simulink model "Wind_Harness"  (R2025b)
settings: Solver=VariableStepAuto  StartTime=0.0  StopTime=5  FixedStep=5e-5  RelTol=1e-3
PostLoadFcn:
  | WindFarmParam;
values from neighbouring files (symbols this model uses):
  base = struct    [WindFarmParam.m]
  pmsm = struct    [WindFarmParam.m]
  Ts = 5E-5    (= 5e-05)    [BESSGFLParam.m]    (also in BESSGFMParam.m; WindFarmParam.m)
  windController = struct    [WindFarmParam.m]
  windSystem = struct    [WindFarmParam.m]
  windTurbine = saveVarsMat.windTurbine    [WindFarmParam.m]
undefined symbols (not defined in the file or in its folder): DiscIntNeverNeededParam, Inertia
libraries: nesl_utility x34, fl_lib x18, ee_lib x18, eeTransforms x6, eeGeneralControl x5, simulink x4, eePwmGenerator x2, eeSinusoidalMeasurementV2 x1, eePmsmCurrentController x1, custom_lib x1
(part 1 of 2)
settings Model: SimulationMode=accelerator  Creator=skota  LastModifiedBy=skota

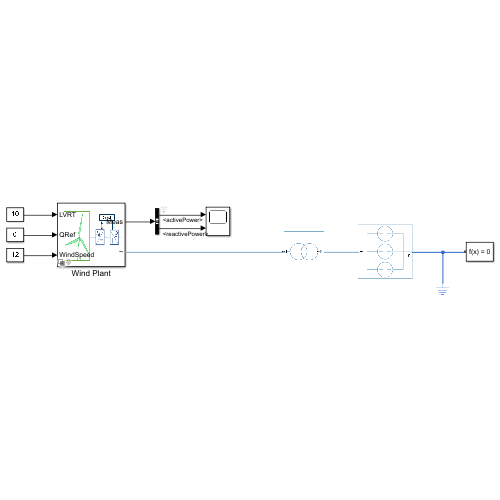
[thumbnail: Simulink's stored preview of the top-level diagram]
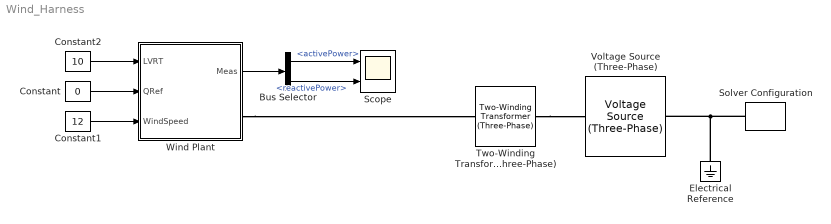
== system Wind_Harness ==
  Bus Selector : BusSelector  OutputSignals=activePower,reactivePower
  Constant : Constant  Value=0
  Constant1 : Constant  Value=12
  Constant2 : Constant  Value=10
  Electrical Reference : fl_lib/Electrical/Electrical Elements/Electrical Reference
  Scope : Scope  NumInputPorts=2
      settings: ActiveDisplayYMinimum=-1.9855696371551242E+9  ActiveDisplayYMaximum=1.7870126734384418E+10
  Solver Configuration : nesl_utility/Solver Configuration  PhysicalDomain=network_engine_domain  SubClassName=solver  LeftPortType=input  RightPortType=generic  Tones=[]  Harmonics=[]  SimulateNoise=off  Profile=off  UseLocalSampling=off  EnableSwitchedLinearOptims=on  FrequencyDomain=off  UseCCode=off  RelTol=0.001  AbsTol=0.001  MinStep=1e-09  ToWorkspace=off  RevertToSquareIcSolve=off  NumHomotopyIterations=100  PhasorMode=off  PhasorModeNumHarmonics=1  ConsistencySolver=NEWTON_XTOL_AFTER_FTOL  IndexReductionMethod=None  DoDC=off  ResidualTolerance=1e-09  ConsistencyTolSource=GLOBAL  ConsistencyAbsTol=0.001  ConsistencyRelTol=0.001  ConsistencyTolFactor=1e-3  UseLocalSolver=on  LocalSolverChoice=NE_BACKWARD_EULER_ADVANCER  ResolveIndetEquations=off  FunctionEvalNumThread=1  LocalSolverSampleTime=Ts  DoFixedCost=on  MaxNonlinIter=1  MaxModeIter=2  ComputeImpulses=off  ImpulseIterations=2  LinearAlgebra=Sparse  LinearAlgebraNumThread=0  EquationFormulation=NE_TIME_EF  DelaysMemoryBudget=1024  AutomaticFiltering=off  FilteringTimeConstant=0.001  PartitionStorageMethod=AS_NEEDED  PartitionMemoryBudget=1024  PartitionMethod=ROBUST  MultibodyUseLocalSolver=off  MultibodyLocalSolverChoice=ODE1  MultibodyLocalSolverSampleTime=0.001
  Two-Winding Transformer (Three-Phase) : ee_lib/Passive/Transformers/Two-Winding Transformer (Three-Phase)  SRated=1000e6 A*V  FRated=50 Hz  Winding1Connection=ee.enum.windingconnection.Yg  VRated1=690 V  Winding2Connection=ee.enum.windingconnection.Yg  VRated2=6600 V  CoreType=ee.enum.coretype.threelimb  pu_Rw1=0.01  pu_Rw2=0.01  leakage_reactance_option=ee.enum.transformer_leakage.include  pu_Xl1=0.05  pu_Xl2=0.05  magnetizing_resistance_option=ee.enum.transformer_magnetizingResistance.include  pu_Rm=500  magnetizing_reactance_option=ee.enum.transformer_magnetizingReactance.include  saturation_option=ee.enum.transformer_saturation.exclude  pu_Xm=500  current_data=[0, .002, 1, 2]  magnetic_flux_data=[0, 1.2, 1.5, 1.51]  pu_X0=0.5  i1_specify=off  i1_priority=None  i1=[0, 0, 0] A  i1_nominal_specify=off  i1_nominal_value=1  i1_nominal_unit=A  i2_specify=off  i2_priority=None  i2=[0, 0, 0] A  i2_nominal_specify=off  i2_nominal_value=1  i2_nominal_unit=A  phi_specify=off  phi_priority=None  phi=[0, 0, 0]  phi_nominal_specify=off  phi_nominal_value=1  phi_nominal_unit=1  power_dissipated_specify=off  power_dissipated_priority=None  power_dissipated=0 W  power_dissipated_nominal_specify=off  power_dissipated_nominal_value=1  power_dissipated_nominal_unit=W
      settings: InternalSimscapePortConfiguration="{\"Bottom\":[],\"Left\":[{\"id\":\"N1\",\"label\":\"~1\",\"type\":\"foundation.electrical.three_phase\"}],\"Right\":[{\"id\":\"N2\",\"label\":\"~2\",\"type\":\"foundation.electrical.three_phase\"}],\"Top\":[]}"
  Voltage Source (Three-Phase) : ee_lib/Sources/Voltage Source (Three-Phase)  vline_rms=6600 V  shift=0 deg  freq=50 Hz  impedance_option=0  SShortCircuit=100e6 A*V  XR=15  R=0.01 Ohm  L=3.97e-4 H  harmonic_option=0  harmonic_orders=[5, 7, 11, 13]  harmonic_ratios=[.1, .1, .1, .1]  G_parasitic=0 1/Ohm  I_specify=off  I_priority=None  I=[0, 0, 0] A  I_nominal_specify=off  I_nominal_value=1  I_nominal_unit=A
  Wind Plant : Subsystem  Variant=on  VariantControlMode=label  LabelModeActiveChoice=Detailed  mask(Wind){fidelity=Detailed, plantRating=windSystem.plantRating, Vac=windSystem.Vac, frequency=windSystem.frequency, iMaxPU=windSystem.iMaxPU, efficiency=windSystem.converterEfficiency, baseVoltageDC=windSystem.Vdc, airDensity=windTurbine.airDensity, turbineRadius=windTurbine.turbineRadius, pitch=windTurbine.pitch, TSR=windTurbine.TSR, cp=windTurbine.cp, wt=windTurbine.wThreshold, rt=windTurbine.wThreshold, p=pmsm.polePairs, psim=pmsm.fluxLinkage, Rs=pmsm.Rs, Ld=pmsm.Ld, Lq=pmsm.Lq, capacitance=windSystem.capacitance, filterInductance=windSystem.filterInductance, filterResistance=windSystem.filterResistance, converterFidelity=Average, fSw=20}
      mask prompts: fidelity "Modeling Option"; plantRating "Wind Farm Rating (kW)"; Vac "Rated AC side voltage (phase-phase RMS) (V)"; frequency "Rated electrical frequency at AC side (Hz)"; iMaxPU "Maximum converter current (pu)"; efficiency "Converter Efficiency (%)"; baseVoltageDC "Voltage on DC side (V)"; airDensity "Air density (kg/m^3)"; turbineRadius "Turbine radius (m)"; pitch "Pitch angle vector (deg)"; TSR "Tip speed ratio"; cp "Power coefficient table, Cp(beta,TSR)"; wt "Wind velocity threshold (m/s)"; rt "Rotational velocity threshold (rad/s)"; p "Number of pole pairs"; psim "PMSM flux linkage (Wb)"; Rs "Stator resistance (Ohm)"; Ld "Stator d-axis inductance (H)"; Lq "Stator q-axis inductance (H)"; capacitance "DC bus capacitance (F)"; filterInductance "Filter inductance (H)"; filterResistance "Filter series resistance (Ohm)"; converterFidelity "Converter Fidelity"; fSw "Switching Frequency (kHz)"
      mask help: This block models a detailed Type -4 ind farm with the MPPT Controller. The wind farm comprises a permanent magnnet synhronous machine connected to the main grid via back-to-back converters. Select simplified mode for faster simulation using fixed efficiency and rated power.
      settings: CopyFcn=set_param(gcbh,'LinkStatus','none');
      mask Help: web('WindFarm.html')
      mask TypeOptions fidelity: Detailed | Simplified
      mask Callback fidelity:
      | detailedTabs = {'windDetailed','controllerDetailed','converter'};
      |     simplifiedTabs = {'windSimplified'};
      |     component.mask.fidelitySelection(detailedTabs,simplifiedTabs);
      mask TypeOptions airDensity: Detailed/Wind System/airDensity
      mask TypeOptions turbineRadius: Detailed/Wind System/turbineRadius
      mask TypeOptions pitch: Detailed/Wind System/pitch
      mask TypeOptions TSR: Detailed/Wind System/TSR
      mask TypeOptions cp: Detailed/Wind System/cp
      mask TypeOptions wt: Detailed/Wind System/wt
      mask TypeOptions rt: Detailed/Wind System/rt
      mask TypeOptions p: Detailed/Wind System/p
      mask TypeOptions psim: Detailed/Wind System/psim
      mask TypeOptions Rs: Detailed/Wind System/Rs
      mask TypeOptions Ld: Detailed/Wind System/Ld
      mask TypeOptions Lq: Detailed/Wind System/Lq
      mask TypeOptions converterFidelity: Detailed/Wind Turbine and Converters/Wind Plant/converterFidelity
      mask Callback converterFidelity:
      | converterFidelity = get_param(gcb,'converterFidelity');
      | blockPath = [gcb,'/','Detailed','/','Wind Turbine and Converters','/','Wind Plant','/','Back-to-Back Converters'];
      | % if strcmp(converterFidelity,'Average')
      | %     blockPath = [gcb,'/','Detailed','/','Wind Turbine and Converters','/','Wind Plant','/','Back-to-Back Converters'];
      | % else
      | %     blockPath = [gcb,'/','Detailed','/','Wind Turbine and Converters','/','Wind Plant','/','Back-to-Back Converters'];
      | % end
      | component.mask.converterFidelity(blockPath)
      mask TypeOptions fSw: Detailed/Wind Turbine and Converters/Wind Plant/fSw
      mask DialogControl generalDetailed Prompt: General
      mask DialogControl windDetailed Prompt: Wind Turbine
      mask DialogControl configureWindTurbine Prompt: Edit wind turbine parameters
      mask DialogControl configureWindTurbine Callback:
      | blockPath = [gcb,'/','Detailed','/','Wind Turbine and Converters','/','Wind Plant','/','Wind Turbine'];
      |     component.mask.openBlock(blockPath);
      mask DialogControl Container10 Prompt: PMSM
      mask DialogControl configurePMSM Prompt: Edit PMSM parameters
      mask DialogControl configurePMSM Callback:
      | blockPath = [gcb,'/','Detailed','/','Wind Turbine and Converters','/','Wind Plant','/','PMSG'];
      |  component.mask.openBlock(blockPath);
      mask DialogControl controllerDetailed Prompt: Controller
      mask DialogControl configureWindController Prompt: Edit Wind Controller
      mask DialogControl configureWindController Callback:
      | blockPath = [gcb,'/','Detailed','/','Wind Turbine and Converters','/','Wind Controller'];
      |     component.mask.openBlock(blockPath);
      mask DialogControl windSimplified Prompt: Wind Turbine
      mask DialogControl editWindFarm Prompt: Edit wind farm
      mask DialogControl editWindFarm Callback:
      | blockPath = [gcb,'/','Simplified','/','Wind farm'];
      | component.mask.openBlock(blockPath);
      mask DialogControl converter Prompt: Converter
      mask DialogControl editMSConverter Prompt: Edit machine side converter parameters
      mask DialogControl editMSConverter Callback:
      | blockFidelity = get_param(gcb,'fidelity');
      | converterFidelity = get_param(gcb,'converterFidelity');
      | if strcmp(converterFidelity,'Average')
      |     blockPath = [gcb,'/',blockFidelity,'/','Wind Turbine and Converters','/','Wind Plant','/','Back-to-Back Converters','/',converterFidelity,'/','Machine Side Converter'];
      | else
      |     blockPath = [gcb,'/',blockFidelity,'/','Wind Turbine and Converters','/','Wind Plant','/','Back-to-Back Converters','/',converterFidelity,'/','Machine Side Converter','/','Converter'];
      | end
      | component.mask.openBlock(blockPath);
      mask DialogControl editGSConverter Prompt: Edit grid side converter parameters
      mask DialogControl editGSConverter Callback:
      | blockFidelity = get_param(gcb,'fidelity');
      | converterFidelity = get_param(gcb,'converterFidelity');
      | if strcmp(converterFidelity,'Average')
      |     blockPath = [gcb,'/',blockFidelity,'/','Wind Turbine and Converters','/','Wind Plant','/','Back-to-Back Converters','/',converterFidelity,'/','Grid Side Converter'];
      | else
      |     blockPath = [gcb,'/',blockFidelity,'/','Wind Turbine and Converters','/','Wind Plant','/','Back-to-Back Converters','/',converterFidelity,'/','Grid Side Converter','/','Converter'];
      | end
      | component.mask.openBlock(blockPath);
      mask Display: image('wind_plant.png');
  wires:
  Constant/1 -> Wind Plant/2(QRef)
  Constant1/1 -> Wind Plant/3(WindSpeed)
  Constant2/1 -> Wind Plant/1(LVRT)
  Wind Plant/1(Meas) -> Bus Selector/1
  Bus Selector/1 -> Scope/1  "<activePower>"
  Bus Selector/2 -> Scope/2  "<reactivePower>"
  connections:
  Electrical Reference/LConn1 -- Solver Configuration/RConn1 -- Voltage Source (Three-Phase)/LConn1
  Wind Plant/RConn1 -- Two-Winding Transformer (Three-Phase)/LConn1
  Two-Winding Transformer (Three-Phase)/RConn1 -- Voltage Source (Three-Phase)/RConn1

== system Wind_Harness/Wind Plant ==
  LVRT : Inport
  QRef : Inport  Port=2
  WindSpeed : Inport  Port=3
  Detailed : Subsystem  VariantControl=Detailed
      settings: CopyFcn=set_param(gcbh,'LinkStatus','none');
  Simplified : Subsystem  VariantControl=Simplified
  ~ : PMIOPort  Side=Right
  Meas : Outport

== system Wind_Harness/Wind Plant/Detailed ==
  LVRT : Inport
  QRef : Inport  Port=2
  WindSpeed : Inport  Port=3
  Constant : Constant  Value=0
  L Filter : ee_lib/Passive/RLC Assemblies/RLC (Three-Phase)  port_option=ee.enum.threePhasePort.composite  component_structure=ee.enum.rlc.structure.L  R=1e-3 Ohm  L=filterInductance H  C=1e-6 F  R_parasitic=0 Ohm  G_parasitic=0 1/Ohm  IL_specify=off  IL_priority=High  IL=[0, 0, 0] A  IL_nominal_specify=off  IL_nominal_value=1  IL_nominal_unit=A  VC_specify=off  VC_priority=High  VC=[0, 0, 0] V  VC_nominal_specify=off  VC_nominal_value=1  VC_nominal_unit=V
      settings: InternalSimscapePortConfiguration="{\"Bottom\":[],\"Left\":[{\"id\":\"N1\",\"label\":\"~1\",\"type\":\"foundation.electrical.three_phase\"}],\"Right\":[{\"id\":\"N2\",\"label\":\"~2\",\"type\":\"foundation.electrical.three_phase\"}],\"Top\":[]}"
  Measurements : Subsystem
  PLL : Subsystem
  Wind Turbine and Converters : Subsystem
  ~ : PMIOPort  Side=Right
  Out Bus Element : Outport  PortName=Meas  Element=activePower
  BusElementOut : Outport  PortName=Meas  Element=reactivePower
  BusElementOut1 : Outport  PortName=Meas  Element=voltage
  BusElementOut2 : Outport  PortName=Meas  Element=current
  wires:
  Measurements/4(I) -> PLL/2(I), BusElementOut2/1
  Measurements/3(V) -> PLL/1(V), BusElementOut1/1
  Measurements/2(Q) -> BusElementOut/1
  Measurements/1(P) -> Out Bus Element/1
  Constant/1 -> Wind Turbine and Converters/1(pitch)
  PLL/1(VI) -> Wind Turbine and Converters/5(VIBus)
  QRef/1 -> Wind Turbine and Converters/4(QRef)
  WindSpeed/1 -> Wind Turbine and Converters/2(Wind_speed)
  LVRT/1 -> Wind Turbine and Converters/3(LVRT)
  connections:
  ~/RConn1 -- Measurements/RConn1
  L Filter/RConn1 -- Measurements/LConn1
  L Filter/LConn1 -- Wind Turbine and Converters/RConn1

== system Wind_Harness/Wind Plant/Simplified ==
  LVRT : Inport
  QRef : Inport  Port=2
  WindSpeed : Inport  Port=3
  Measurements : Subsystem
  PS Constant : fl_lib/Physical Signals/Sources/PS Constant  constant=0 deg
  Simulink-PS Converter : nesl_utility/Simulink-PS Converter  PhysicalDomain=network_engine_domain  SubClassName=ps_input  LeftPortType=input  RightPortType=output  PseudoPeriodic=off  Frequencies=[]  NoiseDistribution=none  NoiseParameters=[]  Unit=1  AffineConversion=off  FilteringAndDerivatives=provide  SimscapeFilterOrder=1  InputFilterTimeConstant=0.001  UdotUserProvided=0
  Terminator : Terminator
  Terminator1 : Terminator
  Wind farm : custom_lib/wind_farm  port_option=ee.enum.threePhasePort.composite  FRated=frequency Hz  VRated=Vac V  IMaxPU=iMaxPU  PlantRating=plantRating*1000 W  modelling_option=ModellingOption.maximumPower  airDensity=airDensity kg/m^3  powercoefficient_option=PowerCoefficient.tableLookUp  TurbineRating=plantRating*1000 W  turbineBlades=3  turbineRadius=turbineRadius m  efficiency=100  vWindRated=12 m/s  cutInSpeed=3 m/s  cutOffSpeed=22 m/s  pitch_TLU=pitch deg  lambda_TLU=TSR  Cp_TLU=cp
      settings: InternalSimscapePortConfiguration="{\"Bottom\":[],\"Left\":[{\"id\":\"vWind\",\"label\":\"V\",\"type\":\"input\"},{\"id\":\"pitch\",\"label\":\"β\",\"type\":\"input\"}],\"Right\":[{\"id\":\"N\",\"label\":\"~\",\"type\":\"foundation.electrical.three_phase\"},{\"id\":\"l\",\"label\":\"I\",\"type\":\"output\"},{\"id\":\"p\",\"label\":\"p\",\"type\":\"output\"}],\"Top\":[]}"
  ~ : PMIOPort  Side=Right
  Out Bus Element : Outport  PortName=Meas  Element=activePower
  BusElementOut : Outport  PortName=Meas  Element=reactivePower
  BusElementOut1 : Outport  PortName=Meas  Element=voltage
  BusElementOut2 : Outport  PortName=Meas  Element=current
  wires:
  Measurements/4(I) -> BusElementOut2/1
  Measurements/3(V) -> BusElementOut1/1
  Measurements/2(Q) -> BusElementOut/1
  Measurements/1(P) -> Out Bus Element/1
  WindSpeed/1 -> Simulink-PS Converter/1
  QRef/1 -> Terminator1/1
  LVRT/1 -> Terminator/1
  connections:
  ~/RConn1 -- Measurements/RConn1
  Wind farm/RConn1 -- Measurements/LConn1
  Wind farm/LConn1 -- Simulink-PS Converter/RConn1
  Wind farm/LConn2 -- PS Constant/RConn1

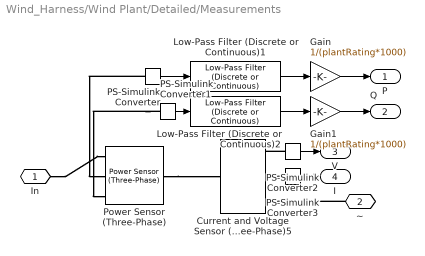
== system Wind_Harness/Wind Plant/Detailed/Measurements ==
  Current and Voltage Sensor (Three-Phase)5 : ee_lib/Sensors & Transducers/Current and Voltage Sensor (Three-Phase)  vMeasurementType=ee.enum.vmeasurement.lg  outputUnit=ee.enum.unit.pu  SRated=plantRating*1000 A*V  VRated=Vac V  I_specify=off  I_priority=None  I=[0, 0, 0] A  I_nominal_specify=off  I_nominal_value=1  I_nominal_unit=A  V_specify=off  V_priority=None  V=[0, 0, 0] V  V_nominal_specify=off  V_nominal_value=1  V_nominal_unit=V
      settings: InternalSimscapePortConfiguration="{\"Bottom\":[],\"Left\":[{\"id\":\"N1\",\"label\":\"~1\",\"type\":\"foundation.electrical.three_phase\"}],\"Right\":[{\"id\":\"V_output\",\"label\":\"V\",\"type\":\"output\"},{\"id\":\"I_output\",\"label\":\"I\",\"type\":\"output\"},{\"id\":\"N2\",\"label\":\"~2\",\"type\":\"foundation.electrical.three_phase\"}],\"Top\":[]}"
  Gain : Gain  Gain=1/(plantRating*1000)
  Gain1 : Gain  Gain=1/(plantRating*1000)
  Low-Pass Filter (Discrete or Continuous)1 : eeGeneralControl/Low-Pass Filter (Discrete or Continuous)  K=1  T=0.1  B=inf  A=-inf  init_option=Inherited from block input  x0=0  Ts=-1
  Low-Pass Filter (Discrete or Continuous)2 : eeGeneralControl/Low-Pass Filter (Discrete or Continuous)  K=1  T=0.1  B=inf  A=-inf  init_option=Inherited from block input  x0=0  Ts=-1
  PS-Simulink Converter{,1..3} (4 alike) : nesl_utility/PS-Simulink Converter  PhysicalDomain=network_engine_domain  SubClassName=ps_output  LeftPortType=input  RightPortType=output  PseudoPeriodic=off  Frequencies=[]  VectorFormat=inherit  Unit=inherit  AffineConversion=off
  Power Sensor (Three-Phase) : ee_lib/Sensors & Transducers/Power Sensor (Three-Phase)  load_type=ee.enum.passive.type_balanced.balanced  f0=60 Hz
      settings: InternalSimscapePortConfiguration="{\"Bottom\":[],\"Left\":[{\"id\":\"N1\",\"label\":\"~1\",\"type\":\"foundation.electrical.three_phase\"}],\"Right\":[{\"id\":\"N2\",\"label\":\"~2\",\"type\":\"foundation.electrical.three_phase\"}],\"Top\":[{\"id\":\"Pm\",\"label\":\"P\",\"type\":\"output\"},{\"id\":\"Qm\",\"label\":\"Q\",\"type\":\"output\"}]}"
  In : PMIOPort  Side=Left
  ~ : PMIOPort  Port=2  Side=Right
  P : Outport
  Q : Outport  Port=2
  V : Outport  Port=3
  I : Outport  Port=4
  wires:
  Gain1/1 -> Q/1
  Gain/1 -> P/1
  PS-Simulink Converter3/1 -> I/1
  PS-Simulink Converter2/1 -> V/1
  Low-Pass Filter (Discrete or Continuous)2/1 -> Gain1/1
  Low-Pass Filter (Discrete or Continuous)1/1 -> Gain/1
  PS-Simulink Converter1/1 -> Low-Pass Filter (Discrete or Continuous)2/1
  PS-Simulink Converter/1 -> Low-Pass Filter (Discrete or Continuous)1/1
  connections:
  PS-Simulink Converter3/LConn1 -- Current and Voltage Sensor (Three-Phase)5/RConn2
  Power Sensor (Three-Phase)/RConn1 -- Current and Voltage Sensor (Three-Phase)5/LConn1
  PS-Simulink Converter1/LConn1 -- Power Sensor (Three-Phase)/LConn3
  ~/RConn1 -- Current and Voltage Sensor (Three-Phase)5/RConn3
  In/RConn1 -- Power Sensor (Three-Phase)/LConn1
  PS-Simulink Converter/LConn1 -- Power Sensor (Three-Phase)/LConn2
  PS-Simulink Converter2/LConn1 -- Current and Voltage Sensor (Three-Phase)5/RConn1

== system Wind_Harness/Wind Plant/Detailed/PLL ==
  V : Inport
  I : Inport  Port=2
  PLL & Measurements1 : Subsystem
  VI : Outport
  wires:
  PLL & Measurements1/1(VIbus) -> VI/1
  I/1 -> PLL & Measurements1/2(I)
  V/1 -> PLL & Measurements1/1(V)

== system Wind_Harness/Wind Plant/Detailed/Wind Turbine and Converters ==
  note: Plant
  note: Controller
  pitch : Inport
  Wind_speed : Inport  Port=2
  LVRT : Inport  Port=3
  QRef : Inport  Port=4
  VIBus : Inport  Port=5
  Signal Conditioning : Subsystem
  Wind Controller : Subsystem  mask(Wind Controller){baseVac=Vac, baseImpedance=Vac^2/(plantRating*1000)%base.impedance, basePower=plantRating*1000, inductance=filterInductance, capacitance=0.1, Vdc=baseVoltageDC, frequency=frequency, iMaxPU=iMaxPU, mpptPower=windSystem.mpptPower, mpptWindSpeed=windSystem.mpptWindSpeed, p=p, psim=psim, Rs=Rs, Ld=Ld, Lq=Lq, airDensity=airDensity, turbineRadius=turbineRadius, pitch=pitch, TSR=TSR, cp=cp, wt=wt, rt=wt, Inertia=200, Kp_dc=windController.kpVoltage, Ki_dc=windController.kiVoltage, Kdpi_g=windController.kpId, Kdii_g=windController.kiId, Kqpi_g=windController.kpIq, Kqii_g=windController.kiIq, Kdip_sm=windController.kpMSC, Kdii_sm=windController.kiMSC, Kqip_sm=windController.kpMSC, Kqii_sm=windController.kiMSC}
      mask prompts: baseVac "Base AC Voltage (V)"; baseImpedance "Base Impedance (Ohm)"; basePower "Base Power (W)"; inductance "Filter Inductance (H)"; capacitance "DC bus capacitance (F)"; Vdc "DC bus Voltage (V)"; frequency "System Frequency (Hz)"; iMaxPU "Maximum Current (pu)"; mpptPower "MPPT Power"; mpptWindSpeed "MPPT Wind Speed"; p "Number of pole pairs"; psim "PMSM flux linkage"; Rs "Stator resistance (Ohm)"; Ld "Stator d-axis inductance (H)"; Lq "Stator q-axis inductance (H)"; airDensity "Air Density (kg/m^3)"; turbineRadius "Turbine radius (m)"; pitch "Pitch angle vector (deg)"; cp "Power Coefficient (cp)"; wt "Wind velocity threshold (m/s)"; rt "Rotational velocity threshold (rad/s)"; Inertia "Turbine Inertia (kgm^2)"; Kp_dc "Proportional gain"; Ki_dc "Integral gain"; Kdpi_g "d-axis proportional gain"; Kdii_g "d-axis integrall gain"; Kqpi_g "q-axis proportional gain"; Kqii_g "q-axis integral gain"; Kdip_sm "d-axis proportional gain"; Kdii_sm "d-axis integral gain"; Kqip_sm "q-axis proportional gain"; Kqii_sm "q-axis integral gain"
      mask help: This block implements the control strategy for a Type-4 wind turbine system, which uses a full-scale back-to-back converter to interface the generator with the grid. The controller manages both the machine-side converter (for generator torque and speed control) and the grid-side converter (for active/reactive power regulation and grid compliance). It ensures smooth power transfer, grid code adherence, and dynamic performance under varying wind and grid conditions. The design supports advanced functionalities such as fault ride-through and voltage support.
      mask DialogControl Container9 Prompt: General
      mask DialogControl Container3 Prompt: PMSM Parameters
      mask DialogControl Container4 Prompt: Wind Turbine Parameters
      mask DialogControl Container6 Prompt: Grid Side Converter Controller
      mask DialogControl Container7 Prompt: DC bus voltage controller
      mask DialogControl Container8 Prompt: Current Controller
      mask DialogControl Container10 Prompt: Machine Side Converter Controller
  Wind Plant : Subsystem  mask(Wind Plant){ratedVoltage=Vac, Vdc=baseVoltageDC, capDC=capacitance, airDensity=airDensity, turbineRadius=turbineRadius, pitch=pitch, TSR=TSR, cp=cp, wt=wt, rt=rt, p=p, psim=psim, Rs=Rs, Ld=Ld, Lq=Lq, converterFidelity=Average, fSw=fSw}
      mask prompts: ratedVoltage "Rated voltage on AC side (V)"; Vdc "DC bus violtage (V)"; capDC "DC bus capacitance (F)"; airDensity "Air density (kg/m^3)"; turbineRadius "Turbine radius (m)"; pitch "Pitch angle vector (deg)"; TSR "Tip speed ratio"; cp "Power coefficient table, Cp(beta,TSR)"; wt "Wind velocity threshold (m/s)"; rt "Rotational velocity threshold (rad/s)"; p "Number of pole pairs"; psim "PMSM flux linkage (Wb)"; Rs "Stator resistance (Ohm)"; Ld "Stator d-axis inductance (H)"; Lq "Stator q-axis inductance (H)"; converterFidelity "Converter Fidelity"; fSw "Switching Frequency (kHz)"
      mask help: This block represents the physical interface between the wind turbine and the power converters. It models the electrical and dynamic characteristics of the wind turbine connected to a converter, while expecting an external control signal for operation
      settings: CopyFcn=set_param(gcbh,'LinkStatus','none');
      mask TypeOptions capDC: Back-to-Back Converters/capDC
      mask TypeOptions converterFidelity: Back-to-Back Converters/converterFidelity
      mask Callback converterFidelity: component.mask.setSwitchingFrequency;
      mask TypeOptions fSw: Back-to-Back Converters/fSw
      mask DialogControl Container4 Prompt: General
      mask DialogControl Container5 Prompt: Wind Turbine
      mask DialogControl editWindTurbine Prompt: Edit Wind Turbine Parameters
      mask DialogControl editWindTurbine Callback:
      | blockPath = [gcb,'/','Wind Turbine'];
      | component.mask.openBlock(blockPath);
      mask DialogControl Container6 Prompt: PMSG
      mask DialogControl editMachine Prompt: Edit PMSG Parameters
      mask DialogControl editMachine Callback:
      | blockPath = [gcb,'/','PMSG'];
      | component.mask.openBlock(blockPath);
      mask DialogControl Container7 Prompt: Converter
      mask DialogControl editMSConverter Prompt: Edit machine side converter parameters
      mask DialogControl editMSConverter Callback:
      | converterFidelity = get_param(gcb,'converterFidelity');
      | if strcmp(converterFidelity,'Average')
      |     blockPath = [gcb,'/','Back-to-Back Converters','/',converterFidelity,'/','Machine Side Converter'];
      | else
      |     blockPath = [gcb,'/','Back-to-Back Converters','/',converterFidelity,'/','Machine Side Converter','/','Converter'];
      | end
      | component.mask.openBlock(blockPath);
      mask DialogControl editGSConverter Prompt: Edit grid side converter parameters
      mask DialogControl editGSConverter Callback:
      | converterFidelity = get_param(gcb,'converterFidelity');
      | if strcmp(converterFidelity,'Average')
      |     blockPath = [gcb,'/','Back-to-Back Converters','/',converterFidelity,'/','Grid Side Converter'];
      | else
      |     blockPath = [gcb,'/','Back-to-Back Converters','/',converterFidelity,'/','Grid Side Converter','/','Converter'];
      | end
      | component.mask.openBlock(blockPath);
      mask Display: image('T4wind.png');
  ~ : PMIOPort  Side=Right
  wires:
  Wind Plant/1(PMSM) -> Signal Conditioning/1(PMSM)
  Wind Plant/2(Meas) -> Signal Conditioning/2(Meas)
  Signal Conditioning/5(windSpeed) -> Wind Controller/5(Wind speed)
  Signal Conditioning/4(Vdc) -> Wind Controller/4(vdc)
  Signal Conditioning/3(theta) -> Wind Controller/3(theta)
  Signal Conditioning/2(rotorSpeed) -> Wind Controller/2(w)
  Signal Conditioning/1(iPMSM) -> Wind Controller/1(iPMSM)
  Wind Controller/1(Chopper Control) -> Wind Plant/3(Chopper)
  pitch/1 -> Wind Plant/1(Pitch)
  Wind_speed/1 -> Wind Plant/2(Wind speed)
  Wind Controller/2(SM converter control) -> Wind Plant/4(Machine)
  Wind Controller/3(m_abc) -> Wind Plant/5(Grid)
  LVRT/1 -> Wind Controller/6(LVRT)
  QRef/1 -> Wind Controller/7(QRef)
  VIBus/1 -> Wind Controller/8(VIbus)
  connections:
  Wind Plant/RConn1 -- ~/RConn1

== system Wind_Harness/Wind Plant/Simplified/Measurements ==
  Current and Voltage Sensor (Three-Phase)5 : ee_lib/Sensors & Transducers/Current and Voltage Sensor (Three-Phase)  vMeasurementType=ee.enum.vmeasurement.lg  outputUnit=ee.enum.unit.pu  SRated=plantRating*1000 A*V  VRated=Vac V  I_specify=off  I_priority=None  I=[0, 0, 0] A  I_nominal_specify=off  I_nominal_value=1  I_nominal_unit=A  V_specify=off  V_priority=None  V=[0, 0, 0] V  V_nominal_specify=off  V_nominal_value=1  V_nominal_unit=V
      settings: InternalSimscapePortConfiguration="{\"Bottom\":[],\"Left\":[{\"id\":\"N1\",\"label\":\"~1\",\"type\":\"foundation.electrical.three_phase\"}],\"Right\":[{\"id\":\"V_output\",\"label\":\"V\",\"type\":\"output\"},{\"id\":\"I_output\",\"label\":\"I\",\"type\":\"output\"},{\"id\":\"N2\",\"label\":\"~2\",\"type\":\"foundation.electrical.three_phase\"}],\"Top\":[]}"
  Gain : Gain  Gain=1/(plantRating*1000)
  Gain1 : Gain  Gain=1/(plantRating*1000)
  Low-Pass Filter (Discrete or Continuous)1 : eeGeneralControl/Low-Pass Filter (Discrete or Continuous)  K=1  T=0.1  B=inf  A=-inf  init_option=Inherited from block input  x0=0  Ts=-1
  Low-Pass Filter (Discrete or Continuous)2 : eeGeneralControl/Low-Pass Filter (Discrete or Continuous)  K=1  T=0.1  B=inf  A=-inf  init_option=Inherited from block input  x0=0  Ts=-1
  PS-Simulink Converter{,1..3} (4 alike) : nesl_utility/PS-Simulink Converter  PhysicalDomain=network_engine_domain  SubClassName=ps_output  LeftPortType=input  RightPortType=output  PseudoPeriodic=off  Frequencies=[]  VectorFormat=inherit  Unit=inherit  AffineConversion=off
  Power Sensor (Three-Phase) : ee_lib/Sensors & Transducers/Power Sensor (Three-Phase)  load_type=ee.enum.passive.type_balanced.balanced  f0=60 Hz
      settings: InternalSimscapePortConfiguration="{\"Bottom\":[],\"Left\":[{\"id\":\"N1\",\"label\":\"~1\",\"type\":\"foundation.electrical.three_phase\"}],\"Right\":[{\"id\":\"N2\",\"label\":\"~2\",\"type\":\"foundation.electrical.three_phase\"}],\"Top\":[{\"id\":\"Pm\",\"label\":\"P\",\"type\":\"output\"},{\"id\":\"Qm\",\"label\":\"Q\",\"type\":\"output\"}]}"
  In : PMIOPort  Side=Left
  ~ : PMIOPort  Port=2  Side=Right
  P : Outport
  Q : Outport  Port=2
  V : Outport  Port=3
  I : Outport  Port=4
  wires:
  Gain1/1 -> Q/1
  Gain/1 -> P/1
  PS-Simulink Converter3/1 -> I/1
  PS-Simulink Converter2/1 -> V/1
  Low-Pass Filter (Discrete or Continuous)2/1 -> Gain1/1
  Low-Pass Filter (Discrete or Continuous)1/1 -> Gain/1
  PS-Simulink Converter1/1 -> Low-Pass Filter (Discrete or Continuous)2/1
  PS-Simulink Converter/1 -> Low-Pass Filter (Discrete or Continuous)1/1
  connections:
  PS-Simulink Converter3/LConn1 -- Current and Voltage Sensor (Three-Phase)5/RConn2
  Power Sensor (Three-Phase)/RConn1 -- Current and Voltage Sensor (Three-Phase)5/LConn1
  PS-Simulink Converter1/LConn1 -- Power Sensor (Three-Phase)/LConn3
  ~/RConn1 -- Current and Voltage Sensor (Three-Phase)5/RConn3
  In/RConn1 -- Power Sensor (Three-Phase)/LConn1
  PS-Simulink Converter/LConn1 -- Power Sensor (Three-Phase)/LConn2
  PS-Simulink Converter2/LConn1 -- Current and Voltage Sensor (Three-Phase)5/RConn1

== system Wind_Harness/Wind Plant/Detailed/PLL/PLL & Measurements1 ==
  V : Inport
  I : Inport  Port=2
  Lead-Lag (Discrete or Continuous) : eeGeneralControl/Lead-Lag (Discrete or Continuous)  T1=0  T2=2e-5  B=inf  A=-inf  init_option=Inherited from block input  x0=0  Ts=Ts
  Subsystem : Subsystem
  Out Bus Element : Outport  PortName=VIbus  Element=Vq
  Out Bus Element1 : Outport  PortName=VIbus  Element=Vd
  Out Bus Element2 : Outport  PortName=VIbus  Element=Freq
  Out Bus Element3 : Outport  PortName=VIbus  Element=Theta
  Out Bus Element4 : Outport  PortName=VIbus  Element=Vmag
  Out Bus Element5 : Outport  PortName=VIbus  Element=Iq
  Out Bus Element6 : Outport  PortName=VIbus  Element=Id
  Out Bus Element7 : Outport  PortName=VIbus  Element=Iabc
  Out Bus Element8 : Outport  PortName=VIbus  Element=Vabc
  wires:
  Lead-Lag (Discrete or Continuous)/1 -> Out Bus Element7/1
  Subsystem/2(freq) -> Out Bus Element2/1
  Subsystem/5(Vq) -> Out Bus Element/1
  Subsystem/3(angle) -> Out Bus Element3/1
  Subsystem/4(Vd) -> Out Bus Element1/1
  V/1 -> Out Bus Element8/1, Subsystem/1(Vabc)
  Subsystem/1(mag) -> Out Bus Element4/1
  I/1 -> Lead-Lag (Discrete or Continuous)/1, Subsystem/2(Iabc)
  Subsystem/7(Iq1) -> Out Bus Element5/1
  Subsystem/6(Id1) -> Out Bus Element6/1

== system Wind_Harness/Wind Plant/Detailed/Wind Turbine and Converters/Signal Conditioning ==
  note: 2
  Bus Element In : Inport  PortName=PMSM  Element=rotorAngle
  BusElementIn2 : Inport  PortName=PMSM  Element=iabc
  BusElementIn3 : Inport  PortName=PMSM  Element=rotorSpeed
  BusElementIn4 : Inport  Port=2  PortName=Meas  Element=windSpeed
  BusElementIn5 : Inport  Port=2  PortName=Meas  Element=Vdc
  Gain : Gain  Gain=-1
  iPMSM : Outport
  rotorSpeed : Outport  Port=2
  theta : Outport  Port=3
  Vdc : Outport  Port=4
  windSpeed : Outport  Port=5
  wires:
  Gain/1 -> iPMSM/1
  BusElementIn2/1 -> Gain/1
  BusElementIn3/1 -> rotorSpeed/1
  Bus Element In/1 -> theta/1
  BusElementIn5/1 -> Vdc/1
  BusElementIn4/1 -> windSpeed/1

== system Wind_Harness/Wind Plant/Detailed/Wind Turbine and Converters/Wind Controller ==
  iPMSM : Inport
  w : Inport  Port=2
  theta : Inport  Port=3
  vdc : Inport  Port=4
  Wind speed : Inport  Port=5
  LVRT : Inport  Port=6
  QRef : Inport  Port=7
  VIbus : Inport  Port=8
  Machine Converter Control : Subsystem
  Wind Grid-side Converter Controller : Subsystem
  Chopper Control : Outport
  SM converter control : Outport  Port=2
  m_abc : Outport  Port=3
  wires:
  Wind Grid-side Converter Controller/1(FRT) -> Machine Converter Control/6(LVRT)
  Wind Grid-side Converter Controller/2(m_abc) -> m_abc/1
  iPMSM/1 -> Machine Converter Control/1(iabc_sens)
  vdc/1 -> Wind Grid-side Converter Controller/4(Vdc), Machine Converter Control/4(vdc_sens)
  Wind speed/1 -> Machine Converter Control/5(Wind speed)
  Machine Converter Control/1(SM converter control) -> SM converter control/1
  theta/1 -> Machine Converter Control/3(a_sens)
  Machine Converter Control/2(Chopper Control) -> Chopper Control/1
  w/1 -> Machine Converter Control/2(w_sens)
  VIbus/1 -> Wind Grid-side Converter Controller/2(VIBus)
  QRef/1 -> Wind Grid-side Converter Controller/1(QRef)
  LVRT/1 -> Wind Grid-side Converter Controller/3(LVRT)

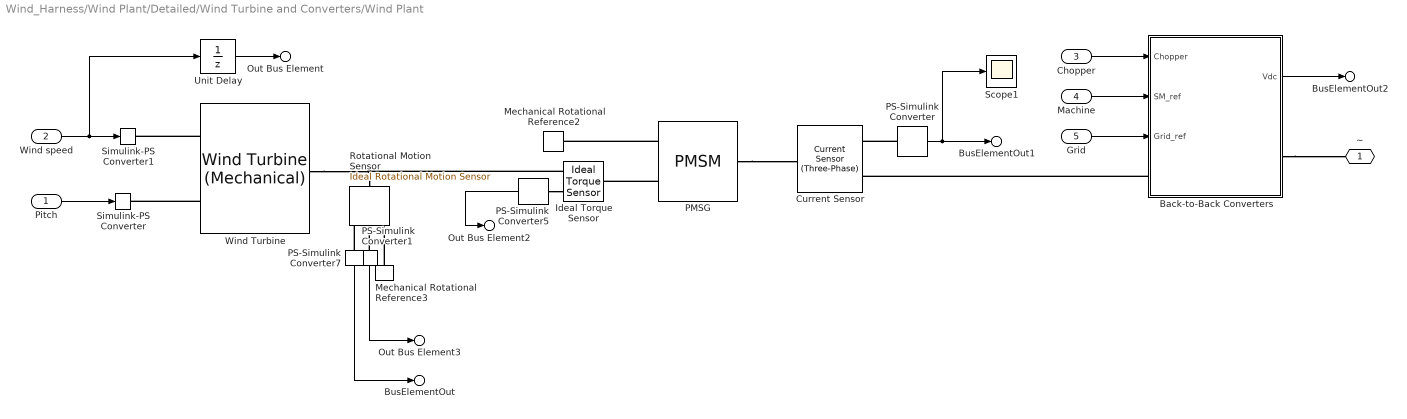
== system Wind_Harness/Wind Plant/Detailed/Wind Turbine and Converters/Wind Plant ==
  Pitch : Inport
  Wind speed : Inport  Port=2
  Chopper : Inport  Port=3
  Machine : Inport  Port=4
  Grid : Inport  Port=5
  Back-to-Back Converters : Subsystem  Variant=on  VariantControlMode=label  LabelModeActiveChoice=Average  mask{converterFidelity=Average, capDC=capDC, fSw=fSw}
      mask prompts: converterFidelity "Converter Fidelity"; capDC "DC bus capacitance (F)"; fSw "Switching Frequency (kHz)"
      settings: CopyFcn=set_param(gcb,'LinkStatus','none');
      mask TypeOptions converterFidelity: Average | Switching
      mask Callback converterFidelity: component.mask.converterFidelity(gcb);
      mask DialogControl editMSConverter Prompt: Edit machine  side converter parameters
      mask DialogControl editMSConverter Callback:
      | converterFidelity = get_param(gcb,'converterFidelity');
      | if strcmp(converterFidelity,'Average')
      |     blockPath = [gcb,'/',converterFidelity,'/','Machine Side Converter'];
      | else
      |     blockPath = [gcb,'/',converterFidelity,'/','Machine Side Converter','/','Converter'];
      | end
      |     component.mask.openConverterBlock(blockPath);
      mask DialogControl editGSConverter Prompt: Edit grid  side converter parameters
      mask DialogControl editGSConverter Callback:
      | converterFidelity = get_param(gcb,'converterFidelity');
      | if strcmp(converterFidelity,'Average')
      |     blockPath = [gcb,'/',converterFidelity,'/','Grid Side Converter'];
      | else
      |     blockPath = [gcb,'/',converterFidelity,'/','Grid Side Converter','/','Converter'];
      | end
      | component.mask.openConverterBlock(blockPath);
  Current Sensor : ee_lib/Sensors & Transducers/Current Sensor (Three-Phase)
  Ideal Torque Sensor : fl_lib/Mechanical/Mechanical Sensors/Ideal Torque Sensor
  Mechanical Rotational Reference2 : fl_lib/Mechanical/Rotational Elements/Mechanical Rotational Reference
  Mechanical Rotational Reference3 : fl_lib/Mechanical/Rotational Elements/Mechanical Rotational Reference
  PMSG : ee_lib/Electromechanical/Permanent Magnet/PMSM  port_option=ee.enum.threePhasePort.composite  winding_type=ee.enum.statorconnection.wye  machine_param=ee.enum.pmsm.parameterization.constant  nPolePairs=p  pmflux_param=ee.enum.pmflux.fluxlinkage  pm_flux_linkage=psim Wb  torque_constant=0.18 N*m/A  back_emf_constant=0.18 V*s/rad  stator_param=ee.enum.statorparam.LdLqL0  Ld=Ld H  Lq=Lq H  idVec=[-200, 0, 200] A  iqVec=[-200, 0, 200] A  LdMatrix=0.0002 * ones(3, 3) H  LqMatrix=0.0002 * ones(3, 3) H  PmMatrix=0.1 * ones(3, 3) Wb  ktMatrix=0.18 * ones(3, 3) N*m/A  keMatrix=0.18 * ones(3, 3) V*s/rad  L0=0.00016 H  Ls=0.0002 H  Lm=-0.00002 H  Ms=0.00002 H  Rs=Rs Ohm  zero_sequence=ee.enum.park.zerosequence.exclude  axes_param=ee.enum.rotorangle.qaxis  loss_param=ee.enum.ironloss.none  losses_oc=[0, 0, 0] W  losses_sc=[0, 0, 0] W  f_losses=60 Hz  Isc_losses=95 A  J=200 kg*m^2  lam=1e-2 N*m*s/rad  i_d_specify=off  i_d_priority=None  i_d=0 A  i_d_nominal_specify=off  i_d_nominal_value=1  i_d_nominal_unit=A  i_q_specify=off  i_q_priority=None  i_q=0 A  i_q_nominal_specify=off  i_q_nominal_value=1  i_q_nominal_unit=A  torque_specify=off  torque_priority=None  torque=0 N*m  torque_nominal_specify=off  torque_nominal_value=1  torque_nominal_unit=N*m  angular_velocity_specify=off  angular_velocity_priority=Low  angular_velocity=2.26 rad/s  angular_velocity_nominal_specify=off  angular_velocity_nominal_value=1  angular_velocity_nominal_unit=rpm  angular_position_specify=off  angular_position_priority=High  angular_position=0 deg  angular_position_nominal_specify=off  angular_position_nominal_value=1  angular_position_nominal_unit=deg  alpha=3.93e-3 1/K  alpha_flux=-0.001 1/K  Tmeas=298.15 K  stator_thermal_mass=100 J/K  rotor_thermal_mass=200 J/K  Rm_percent_rotor=90  Rd_percent_rotor=30  temperatureA_specify=off  temperatureA_priority=High  temperatureA=25 degC  temperatureA_nominal_specify=off  temperatureA_nominal_value=1  temperatureA_nominal_unit=degC  temperatureB_specify=off  temperatureB_priority=High  temperatureB=25 degC  temperatureB_nominal_specify=off  temperatureB_nominal_value=1  temperatureB_nominal_unit=degC  temperatureC_specify=off  temperatureC_priority=High  temperatureC=25 degC  temperatureC_nominal_specify=off  temperatureC_nominal_value=1  temperatureC_nominal_unit=degC  temperatureR_specify=off  temperatureR_priority=High  temperatureR=25 degC  temperatureR_nominal_specify=off  temperatureR_nominal_value=1  temperatureR_nominal_unit=degC
      settings: InternalSimscapePortConfiguration="{\"Bottom\":[],\"Left\":[{\"id\":\"N\",\"label\":\"~\",\"type\":\"foundation.electrical.three_phase\"}],\"Right\":[{\"id\":\"R\",\"label\":\"R\",\"type\":\"foundation.mechanical.rotational.rotational\"},{\"id\":\"C\",\"label\":\"C\",\"type\":\"foundation.mechanical.rotational.rotational\"}],\"Top\":[]}"
  PS-Simulink Converter : nesl_utility/PS-Simulink Converter  PhysicalDomain=network_engine_domain  SubClassName=ps_output  LeftPortType=input  RightPortType=output  PseudoPeriodic=off  Frequencies=[]  VectorFormat=1-D array  Unit=A  AffineConversion=off
  PS-Simulink Converter1 : nesl_utility/PS-Simulink Converter  PhysicalDomain=network_engine_domain  SubClassName=ps_output  LeftPortType=input  RightPortType=output  PseudoPeriodic=off  Frequencies=[]  VectorFormat=inherit  Unit=rad/s  AffineConversion=off
  PS-Simulink Converter5 : nesl_utility/PS-Simulink Converter  PhysicalDomain=network_engine_domain  SubClassName=ps_output  LeftPortType=input  RightPortType=output  PseudoPeriodic=off  Frequencies=[]  VectorFormat=1-D array  Unit=N*m  AffineConversion=off
  PS-Simulink Converter7 : nesl_utility/PS-Simulink Converter  PhysicalDomain=network_engine_domain  SubClassName=ps_output  LeftPortType=input  RightPortType=output  PseudoPeriodic=off  Frequencies=[]  VectorFormat=1-D array  Unit=rad  AffineConversion=off
  Rotational Motion Sensor : fl_lib/Mechanical/Mechanical Sensors/Ideal Rotational Motion Sensor  reference=foundation.enum.MeasurementReference.difference  acceleration_port=false  velocity_port=true  position_port=true  wrap_angle=simscape.enum.onoff.off  offset=0 deg
  Scope1 : Scope
      settings: ActiveDisplayYMinimum=-6255.05498425373  ActiveDisplayYMaximum=6362.825931701329  DataLoggingVariableName=ScopeData6
  Simulink-PS Converter : nesl_utility/Simulink-PS Converter  PhysicalDomain=network_engine_domain  SubClassName=ps_input  LeftPortType=input  RightPortType=output  PseudoPeriodic=off  Frequencies=[]  NoiseDistribution=none  NoiseParameters=[]  Unit=1  AffineConversion=off  FilteringAndDerivatives=provide  SimscapeFilterOrder=1  InputFilterTimeConstant=0.001  UdotUserProvided=0
  Simulink-PS Converter1 : nesl_utility/Simulink-PS Converter  PhysicalDomain=network_engine_domain  SubClassName=ps_input  LeftPortType=input  RightPortType=output  PseudoPeriodic=off  Frequencies=[]  NoiseDistribution=none  NoiseParameters=[]  Unit=1  AffineConversion=off  FilteringAndDerivatives=provide  SimscapeFilterOrder=1  InputFilterTimeConstant=0.001  UdotUserProvided=0
  Unit Delay : UnitDelay  SampleTime=-1  HasFrameUpgradeWarning=on
  Wind Turbine : ee_lib/Electromechanical/Wind Turbine (Mechanical)  R_rotor=turbineRadius m  pitch_TLU=pitch deg  lambda_TLU=TSR  Cp_TLU=cp  v_thr=wt m/s  w_thr=rt rad/s  rho_air=airDensity kg/m^3  includeInertia=false  J=Inertia kg*m^2  lam=10 N*m*s/rad  w_specify=off  w_priority=Low  w=2.262*2.5 rad/s  w_nominal_specify=off  w_nominal_value=1  w_nominal_unit=rad/s  t_specify=off  t_priority=None  t=0 N*m  t_nominal_specify=off  t_nominal_value=1  t_nominal_unit=N*m  Torque_specify=off  Torque_priority=None  Torque=0 N*m  Torque_nominal_specify=off  Torque_nominal_value=1  Torque_nominal_unit=N*m
      settings: InternalSimscapePortConfiguration="{\"Bottom\":[],\"Left\":[{\"id\":\"vWind\",\"label\":\"V\",\"type\":\"input\"},{\"id\":\"pitch\",\"label\":\"β\",\"type\":\"input\"}],\"Right\":[{\"id\":\"R\",\"label\":\"R\",\"type\":\"foundation.mechanical.rotational.rotational\"}],\"Top\":[]}"
  ~ : PMIOPort  Side=Right
  Out Bus Element2 : Outport  PortName=PMSM  Element=torque
  Out Bus Element3 : Outport  PortName=PMSM  Element=rotorSpeed
  BusElementOut : Outport  PortName=PMSM  Element=rotorAngle
  BusElementOut1 : Outport  PortName=PMSM  Element=iabc
  Out Bus Element : Outport  Port=2  PortName=Meas  Element=windSpeed
  BusElementOut2 : Outport  Port=2  PortName=Meas  Element=Vdc
  wires:
  Back-to-Back Converters/1(Vdc) -> BusElementOut2/1
  Machine/1 -> Back-to-Back Converters/2(SM_ref)
  PS-Simulink Converter5/1 -> Out Bus Element2/1
  Wind speed/1 -> Simulink-PS Converter1/1, Unit Delay/1
  PS-Simulink Converter/1 -> BusElementOut1/1, Scope1/1
  Unit Delay/1 -> Out Bus Element/1
  Pitch/1 -> Simulink-PS Converter/1
  PS-Simulink Converter1/1 -> Out Bus Element3/1
  Chopper/1 -> Back-to-Back Converters/1(Chopper)
  Grid/1 -> Back-to-Back Converters/3(Grid_ref)
  PS-Simulink Converter7/1 -> BusElementOut/1
  connections:
  Wind Turbine/LConn1 -- Simulink-PS Converter1/RConn1
  Wind Turbine/LConn2 -- Simulink-PS Converter/RConn1
  Back-to-Back Converters/LConn1 -- Current Sensor/RConn2
  PS-Simulink Converter5/LConn1 -- Ideal Torque Sensor/RConn2
  Mechanical Rotational Reference3/LConn1 -- Rotational Motion Sensor/RConn1
  PMSG/RConn1 -- Ideal Torque Sensor/LConn1
  Rotational Motion Sensor/LConn1 -- Wind Turbine/RConn1 -- Ideal Torque Sensor/RConn1
  PMSG/RConn2 -- Mechanical Rotational Reference2/LConn1
  PMSG/LConn1 -- Current Sensor/LConn1
  PS-Simulink Converter1/LConn1 -- Rotational Motion Sensor/RConn2
  PS-Simulink Converter7/LConn1 -- Rotational Motion Sensor/RConn3
  Back-to-Back Converters/RConn1 -- ~/RConn1
  PS-Simulink Converter/LConn1 -- Current Sensor/RConn1

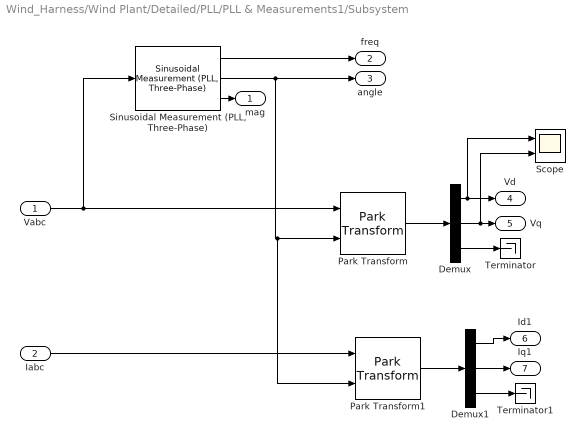
== system Wind_Harness/Wind Plant/Detailed/PLL/PLL & Measurements1/Subsystem ==
  Vabc : Inport
  Iabc : Inport  Port=2
  Demux : Demux  Outputs=3
  Demux1 : Demux  Outputs=3
  Park Transform : eeTransforms/Park Transform  AxisAlignment=Q-axis  PowerInvariant=off
  Park Transform1 : eeTransforms/Park Transform  AxisAlignment=Q-axis  PowerInvariant=off
  Scope : Scope  NumInputPorts=2
      settings: ActiveDisplayYMinimum=0.95416  ActiveDisplayYMaximum=1.02793  DataLoggingVariableName=ScopeData5
  "Sinusoidal Measurement (PLL, Three-Phase)" : eeSinusoidalMeasurementV2/Sinusoidal Measurement (PLL, Three-Phase)  InputFilter=on  InputNormalization=off  Kp_LF=100  Ki_LF=2000  F0=50  Theta0=0  Ts=Ts
  Terminator : Terminator
  Terminator1 : Terminator
  mag : Outport
  freq : Outport  Port=2
  angle : Outport  Port=3
  Vd : Outport  Port=4
  Vq : Outport  Port=5
  Id1 : Outport  Port=6
  Iq1 : Outport  Port=7
  wires:
  Demux/3 -> Terminator/1
  Vabc/1 -> Park Transform/1, "Sinusoidal Measurement (PLL, Three-Phase)"/1
  Park Transform/1 -> Demux/1
  Demux/1 -> Scope/1, Vd/1
  Demux/2 -> Scope/2, Vq/1
  "Sinusoidal Measurement (PLL, Three-Phase)"/2 -> angle/1, Park Transform1/2, Park Transform/2
  "Sinusoidal Measurement (PLL, Three-Phase)"/1 -> freq/1
  "Sinusoidal Measurement (PLL, Three-Phase)"/3 -> mag/1
  Park Transform1/1 -> Demux1/1
  Demux1/1 -> Id1/1
  Demux1/2 -> Iq1/1
  Demux1/3 -> Terminator1/1
  Iabc/1 -> Park Transform1/1

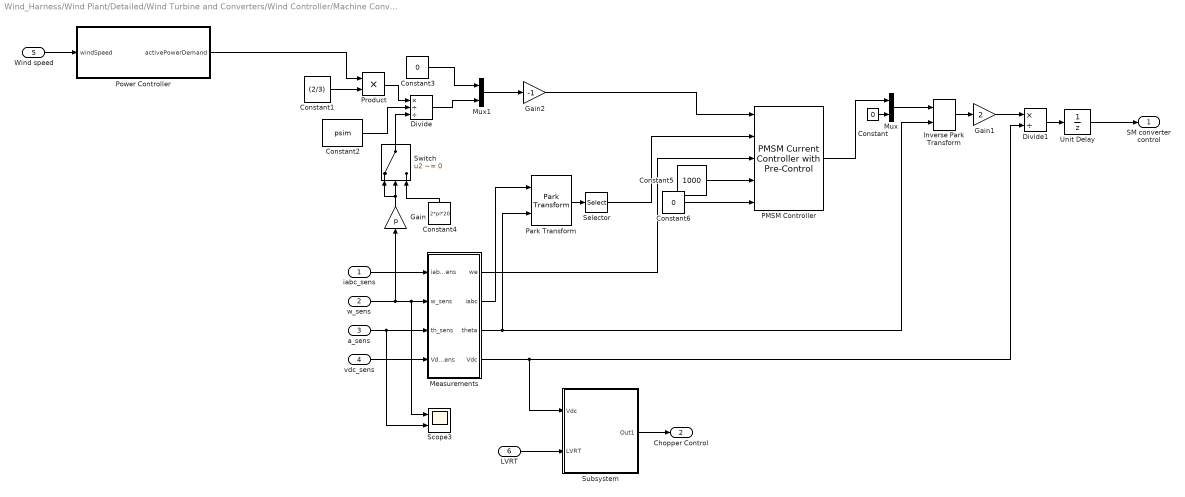
== system Wind_Harness/Wind Plant/Detailed/Wind Turbine and Converters/Wind Controller/Machine Converter Control ==
  iabc_sens : Inport
  w_sens : Inport  Port=2
  a_sens : Inport  Port=3
  vdc_sens : Inport  Port=4
  Wind speed : Inport  Port=5
  LVRT : Inport  Port=6
  Constant : Constant  Value=0  SampleTime=-1
  Constant1 : Constant  Value=(2/3)
  Constant2 : Constant  Value=psim
  Constant3 : Constant  Value=0
  Constant4 : Constant  Value=2*pi*20
  Constant5 : Constant  Value=1000  VectorParams1D=off  SampleTime=-1
  Constant6 : Constant  Value=0
  Divide : Product  Inputs=*//
  Divide1 : Product  Inputs=*/
  Gain : Gain  Gain=p
  Gain1 : Gain  Gain=2
  Gain2 : Gain  Gain=-1
  Inverse Park Transform : eeTransforms/Inverse Park Transform  AxisAlignment=Q-axis  PowerInvariant=off
  Measurements : Subsystem
  Mux : Mux  Inputs=2
  Mux1 : Mux  Inputs=2
  PMSM Controller : eePmsmCurrentController/PMSM Current Controller with Pre-Control  Kp_id=Kdip_sm  Ki_id=Kdii_sm  Kaw_id=0  Kp_iq=Kqip_sm  Ki_iq=Kqii_sm  Kaw_iq=0  Ts=-1  Tsd=0.001  AxisPrio=Q-axis  ActZC=off  ActFF=on  idVect=[-1, 0, 1]  iqVect=[-2000, 0, 2000]  LdMatrix=Ld* ones(3, 3)  LqMatrix=Lq* ones(3, 3)  psimMatrix=psim * ones(3, 3)
  Park Transform : eeTransforms/Park Transform  AxisAlignment=Q-axis  PowerInvariant=off
  Power Controller : Subsystem
  Product : Product
  Scope3 : Scope  NumInputPorts=2
      settings: ActiveDisplayYMinimum=-0.53154558960654574  ActiveDisplayYMaximum=3.2068078785969831  DataLoggingVariableName=ScopeData23
  Selector : Selector  InputPortWidth=3  IndexOptions=Index vector (dialog)  Indices=[1 2]  OutputSizes=1
  Subsystem : Subsystem
  Switch : Switch  Criteria=u2 ~= 0  SaturateOnIntegerOverflow=off  InputSameDT=off
  Unit Delay : UnitDelay  SampleTime=-1  HasFrameUpgradeWarning=on
  SM converter control : Outport  VectorParamsAs1DForOutWhenUnconnected=off
  Chopper Control : Outport  Port=2
  wires:
  Measurements/3(theta) -> Inverse Park Transform/2, Park Transform/2
  w_sens/1 -> Measurements/2(w_sens), Scope3/1, Gain/1
  a_sens/1 -> Measurements/3(th_sens), Scope3/2
  Constant3/1 -> Mux1/1
  Gain/1 -> Switch/2, Switch/1
  Subsystem/1(Out1) -> Chopper Control/1
  Constant5/1 -> PMSM Controller/4
  vdc_sens/1 -> Measurements/4(Vdc_sens)
  Measurements/4(Vdc) -> Divide1/2, Subsystem/1(Vdc)
  Gain2/1 -> PMSM Controller/1
  Mux/1 -> Inverse Park Transform/1
  Inverse Park Transform/1 -> Gain1/1
  Switch/1 -> Divide/3
  Constant6/1 -> PMSM Controller/5
  Measurements/2(iabc) -> Park Transform/1
  Constant/1 -> Mux/2
  iabc_sens/1 -> Measurements/1(iabc_sens)
  Park Transform/1 -> Selector/1
  Constant1/1 -> Product/2
  Constant2/1 -> Divide/2
  Divide1/1 -> Unit Delay/1
  Power Controller/1(activePowerDemand) -> Product/1
  Mux1/1 -> Gain2/1
  PMSM Controller/1 -> Mux/1
  Gain1/1 -> Divide1/1
  Constant4/1 -> Switch/3
  Divide/1 -> Mux1/2
  LVRT/1 -> Subsystem/2(LVRT)
  Selector/1 -> PMSM Controller/2
  Wind speed/1 -> Power Controller/1(windSpeed)
  Unit Delay/1 -> SM converter control/1
  Measurements/1(we) -> PMSM Controller/3
  Product/1 -> Divide/1

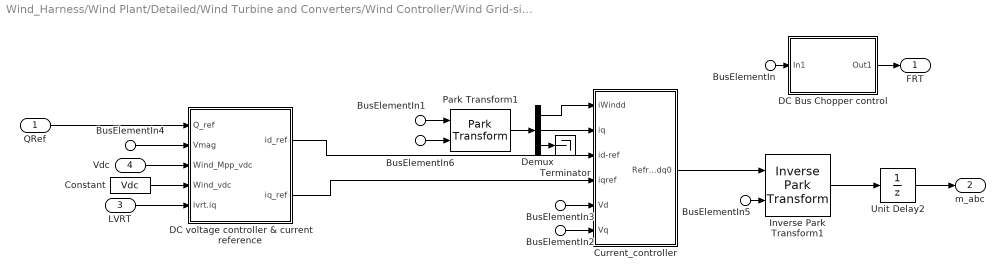
== system Wind_Harness/Wind Plant/Detailed/Wind Turbine and Converters/Wind Controller/Wind Grid-side Converter Controller ==
  QRef : Inport
  BusElementIn : Inport  Port=2  PortName=VIBus  Element=Vmag
  BusElementIn4 : Inport  Port=2  PortName=VIBus  Element=Vmag
  BusElementIn1 : Inport  Port=2  PortName=VIBus  Element=Iabc
  BusElementIn2 : Inport  Port=2  PortName=VIBus  Element=Vq
  BusElementIn3 : Inport  Port=2  PortName=VIBus  Element=Vd
  BusElementIn5 : Inport  Port=2  PortName=VIBus  Element=Theta
  BusElementIn6 : Inport  Port=2  PortName=VIBus  Element=Theta
  LVRT : Inport  Port=3
  Vdc : Inport  Port=4
  Constant : Constant  Value=Vdc
  Current_controller : Subsystem
  "DC Bus Chopper control " : Subsystem
  DC voltage controller & current reference : Subsystem
  Demux : Demux  Outputs=3
  Inverse Park Transform1 : eeTransforms/Inverse Park Transform  AxisAlignment=Q-axis  PowerInvariant=off
  Park Transform1 : eeTransforms/Park Transform  AxisAlignment=Q-axis  PowerInvariant=off
  Terminator : Terminator
  Unit Delay2 : UnitDelay  SampleTime=Ts  HasFrameUpgradeWarning=on
  FRT : Outport
  m_abc : Outport  Port=2
  wires:
  Constant/1 -> DC voltage controller & current reference/4(Wind_vdc)
  Vdc/1 -> DC voltage controller & current reference/3(Wind_Mpp_vdc)
  Demux/3 -> Terminator/1
  "DC Bus Chopper control "/1(Out1) -> FRT/1
  BusElementIn/1 -> "DC Bus Chopper control "/1(In1)
  QRef/1 -> DC voltage controller & current reference/1(Q_ref)
  LVRT/1 -> DC voltage controller & current reference/5(lvrt.iq)
  BusElementIn4/1 -> DC voltage controller & current reference/2(Vmag)
  BusElementIn5/1 -> Inverse Park Transform1/2
  BusElementIn6/1 -> Park Transform1/2
  Current_controller/1(Refrence_mdq0) -> Inverse Park Transform1/1
  Unit Delay2/1 -> m_abc/1
  Inverse Park Transform1/1 -> Unit Delay2/1
  BusElementIn2/1 -> Current_controller/6(Vq)
  Park Transform1/1 -> Demux/1
  Demux/1 -> Current_controller/1(iWindd)
  Demux/2 -> Current_controller/2(iq)
  DC voltage controller & current reference/1(id_ref) -> Current_controller/3(id-ref)
  DC voltage controller & current reference/2(iq_ref) -> Current_controller/4(iqref)
  BusElementIn1/1 -> Park Transform1/1
  BusElementIn3/1 -> Current_controller/5(Vd)
